simulink model "xEMU_SimulationModel3_rule1"  (R2017b)
settings: Solver=ode4  StartTime=0.0  StopTime=8192  FixedStep=0.01  RelTol=1e-3
undefined symbols (not defined in the file): a1, a2, a3, a4, ACO, BAT, Battery, DCT, DRT, EMS, ENV, Fahrzyklus_VS_modell, height_BAT, leistung, lib_bat, Maximum, Maximum_position, Num_cells, P_FC_max_long, P_FC_min_long, P_FC_step_max, Pbat_charge_max, Pbat_discharge_max, Pfc_max, Pfc_min, SOC_tar, time_peaks, TRM, velocity_peaks
libraries: simulink x5
(part 5 of 15)

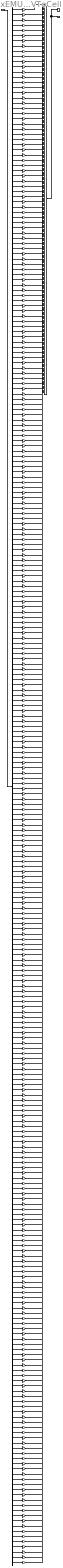
== system xEMU_SimulationModel3_rule1/Battery (BAT)_komplex/Subsystem/Thermal/FVToCell ==
  T_FV : Inport
  AddCell1 : Sum  Inputs=<binary blob, 300 chars, not shown>
  Demux : Demux  Outputs=300
  T_FV_{1..300} (300 alike) : Gain  Gain=0.0033333  SaturateOnIntegerOverflow=on  OutDataTypeStr=Inherit: Same as input  ParamDataTypeStr=Inherit: Same as input
  Out1 : Outport
  tag scope: T_CellElement1=global
  wires:
  T_FV/1 -> Demux/1
  Demux/1 -> T_FV_1/1
  Demux/2 -> T_FV_2/1
  Demux/3 -> T_FV_3/1
  Demux/4 -> T_FV_4/1
  Demux/5 -> T_FV_5/1
  Demux/6 -> T_FV_6/1
  Demux/7 -> T_FV_7/1
  Demux/8 -> T_FV_8/1
  Demux/9 -> T_FV_9/1
  Demux/10 -> T_FV_10/1
  Demux/11 -> T_FV_11/1
  Demux/12 -> T_FV_12/1
  Demux/13 -> T_FV_13/1
  Demux/14 -> T_FV_14/1
  Demux/15 -> T_FV_15/1
  Demux/16 -> T_FV_16/1
  Demux/17 -> T_FV_17/1
  Demux/18 -> T_FV_18/1
  Demux/19 -> T_FV_19/1
  Demux/20 -> T_FV_20/1
  Demux/21 -> T_FV_21/1
  Demux/22 -> T_FV_22/1
  Demux/23 -> T_FV_23/1
  Demux/24 -> T_FV_24/1
  Demux/25 -> T_FV_25/1
  Demux/26 -> T_FV_26/1
  Demux/27 -> T_FV_27/1
  Demux/28 -> T_FV_28/1
  Demux/29 -> T_FV_29/1
  Demux/30 -> T_FV_30/1
  Demux/31 -> T_FV_31/1
  Demux/32 -> T_FV_32/1
  Demux/33 -> T_FV_33/1
  Demux/34 -> T_FV_34/1
  Demux/35 -> T_FV_35/1
  Demux/36 -> T_FV_36/1
  Demux/37 -> T_FV_37/1
  Demux/38 -> T_FV_38/1
  Demux/39 -> T_FV_39/1
  Demux/40 -> T_FV_40/1
  Demux/41 -> T_FV_41/1
  Demux/42 -> T_FV_42/1
  Demux/43 -> T_FV_43/1
  Demux/44 -> T_FV_44/1
  Demux/45 -> T_FV_45/1
  Demux/46 -> T_FV_46/1
  Demux/47 -> T_FV_47/1
  Demux/48 -> T_FV_48/1
  Demux/49 -> T_FV_49/1
  Demux/50 -> T_FV_50/1
  Demux/51 -> T_FV_51/1
  Demux/52 -> T_FV_52/1
  Demux/53 -> T_FV_53/1
  Demux/54 -> T_FV_54/1
  Demux/55 -> T_FV_55/1
  Demux/56 -> T_FV_56/1
  Demux/57 -> T_FV_57/1
  Demux/58 -> T_FV_58/1
  Demux/59 -> T_FV_59/1
  Demux/60 -> T_FV_60/1
  Demux/61 -> T_FV_61/1
  Demux/62 -> T_FV_62/1
  Demux/63 -> T_FV_63/1
  Demux/64 -> T_FV_64/1
  Demux/65 -> T_FV_65/1
  Demux/66 -> T_FV_66/1
  Demux/67 -> T_FV_67/1
  Demux/68 -> T_FV_68/1
  Demux/69 -> T_FV_69/1
  Demux/70 -> T_FV_70/1
  Demux/71 -> T_FV_71/1
  Demux/72 -> T_FV_72/1
  Demux/73 -> T_FV_73/1
  Demux/74 -> T_FV_74/1
  Demux/75 -> T_FV_75/1
  Demux/76 -> T_FV_76/1
  Demux/77 -> T_FV_77/1
  Demux/78 -> T_FV_78/1
  Demux/79 -> T_FV_79/1
  Demux/80 -> T_FV_80/1
  Demux/81 -> T_FV_81/1
  Demux/82 -> T_FV_82/1
  Demux/83 -> T_FV_83/1
  Demux/84 -> T_FV_84/1
  Demux/85 -> T_FV_85/1
  Demux/86 -> T_FV_86/1
  Demux/87 -> T_FV_87/1
  Demux/88 -> T_FV_88/1
  Demux/89 -> T_FV_89/1
  Demux/90 -> T_FV_90/1
  Demux/91 -> T_FV_91/1
  Demux/92 -> T_FV_92/1
  Demux/93 -> T_FV_93/1
  Demux/94 -> T_FV_94/1
  Demux/95 -> T_FV_95/1
  Demux/96 -> T_FV_96/1
  Demux/97 -> T_FV_97/1
  Demux/98 -> T_FV_98/1
  Demux/99 -> T_FV_99/1
  Demux/100 -> T_FV_100/1
  Demux/101 -> T_FV_101/1
  Demux/102 -> T_FV_102/1
  Demux/103 -> T_FV_103/1
  Demux/104 -> T_FV_104/1
  Demux/105 -> T_FV_105/1
  Demux/106 -> T_FV_106/1
  Demux/107 -> T_FV_107/1
  Demux/108 -> T_FV_108/1
  Demux/109 -> T_FV_109/1
  Demux/110 -> T_FV_110/1
  Demux/111 -> T_FV_111/1
  Demux/112 -> T_FV_112/1
  Demux/113 -> T_FV_113/1
  Demux/114 -> T_FV_114/1
  Demux/115 -> T_FV_115/1
  Demux/116 -> T_FV_116/1
  Demux/117 -> T_FV_117/1
  Demux/118 -> T_FV_118/1
  Demux/119 -> T_FV_119/1
  Demux/120 -> T_FV_120/1
  Demux/121 -> T_FV_121/1
  Demux/122 -> T_FV_122/1
  Demux/123 -> T_FV_123/1
  Demux/124 -> T_FV_124/1
  Demux/125 -> T_FV_125/1
  Demux/126 -> T_FV_126/1
  Demux/127 -> T_FV_127/1
  Demux/128 -> T_FV_128/1
  Demux/129 -> T_FV_129/1
  Demux/130 -> T_FV_130/1
  Demux/131 -> T_FV_131/1
  Demux/132 -> T_FV_132/1
  Demux/133 -> T_FV_133/1
  Demux/134 -> T_FV_134/1
  Demux/135 -> T_FV_135/1
  Demux/136 -> T_FV_136/1
  Demux/137 -> T_FV_137/1
  Demux/138 -> T_FV_138/1
  Demux/139 -> T_FV_139/1
  Demux/140 -> T_FV_140/1
  Demux/141 -> T_FV_141/1
  Demux/142 -> T_FV_142/1
  Demux/143 -> T_FV_143/1
  Demux/144 -> T_FV_144/1
  Demux/145 -> T_FV_145/1
  Demux/146 -> T_FV_146/1
  Demux/147 -> T_FV_147/1
  Demux/148 -> T_FV_148/1
  Demux/149 -> T_FV_149/1
  Demux/150 -> T_FV_150/1
  Demux/151 -> T_FV_151/1
  Demux/152 -> T_FV_152/1
  Demux/153 -> T_FV_153/1
  Demux/154 -> T_FV_154/1
  Demux/155 -> T_FV_155/1
  Demux/156 -> T_FV_156/1
  Demux/157 -> T_FV_157/1
  Demux/158 -> T_FV_158/1
  Demux/159 -> T_FV_159/1
  Demux/160 -> T_FV_160/1
  Demux/161 -> T_FV_161/1
  Demux/162 -> T_FV_162/1
  Demux/163 -> T_FV_163/1
  Demux/164 -> T_FV_164/1
  Demux/165 -> T_FV_165/1
  Demux/166 -> T_FV_166/1
  Demux/167 -> T_FV_167/1
  Demux/168 -> T_FV_168/1
  Demux/169 -> T_FV_169/1
  Demux/170 -> T_FV_170/1
  Demux/171 -> T_FV_171/1
  Demux/172 -> T_FV_172/1
  Demux/173 -> T_FV_173/1
  Demux/174 -> T_FV_174/1
  Demux/175 -> T_FV_175/1
  Demux/176 -> T_FV_176/1
  Demux/177 -> T_FV_177/1
  Demux/178 -> T_FV_178/1
  Demux/179 -> T_FV_179/1
  Demux/180 -> T_FV_180/1
  Demux/181 -> T_FV_181/1
  Demux/182 -> T_FV_182/1
  Demux/183 -> T_FV_183/1
  Demux/184 -> T_FV_184/1
  Demux/185 -> T_FV_185/1
  Demux/186 -> T_FV_186/1
  Demux/187 -> T_FV_187/1
  Demux/188 -> T_FV_188/1
  Demux/189 -> T_FV_189/1
  Demux/190 -> T_FV_190/1
  Demux/191 -> T_FV_191/1
  Demux/192 -> T_FV_192/1
  Demux/193 -> T_FV_193/1
  Demux/194 -> T_FV_194/1
  Demux/195 -> T_FV_195/1
  Demux/196 -> T_FV_196/1
  Demux/197 -> T_FV_197/1
  Demux/198 -> T_FV_198/1
  Demux/199 -> T_FV_199/1
  Demux/200 -> T_FV_200/1
  Demux/201 -> T_FV_201/1
  Demux/202 -> T_FV_202/1
  Demux/203 -> T_FV_203/1
  Demux/204 -> T_FV_204/1
  Demux/205 -> T_FV_205/1
  Demux/206 -> T_FV_206/1
  Demux/207 -> T_FV_207/1
  Demux/208 -> T_FV_208/1
  Demux/209 -> T_FV_209/1
  Demux/210 -> T_FV_210/1
  Demux/211 -> T_FV_211/1
  Demux/212 -> T_FV_212/1
  Demux/213 -> T_FV_213/1
  Demux/214 -> T_FV_214/1
  Demux/215 -> T_FV_215/1
  Demux/216 -> T_FV_216/1
  Demux/217 -> T_FV_217/1
  Demux/218 -> T_FV_218/1
  Demux/219 -> T_FV_219/1
  Demux/220 -> T_FV_220/1
  Demux/221 -> T_FV_221/1
  Demux/222 -> T_FV_222/1
  Demux/223 -> T_FV_223/1
  Demux/224 -> T_FV_224/1
  Demux/225 -> T_FV_225/1
  Demux/226 -> T_FV_226/1
  Demux/227 -> T_FV_227/1
  Demux/228 -> T_FV_228/1
  Demux/229 -> T_FV_229/1
  Demux/230 -> T_FV_230/1
  Demux/231 -> T_FV_231/1
  Demux/232 -> T_FV_232/1
  Demux/233 -> T_FV_233/1
  Demux/234 -> T_FV_234/1
  Demux/235 -> T_FV_235/1
  Demux/236 -> T_FV_236/1
  Demux/237 -> T_FV_237/1
  Demux/238 -> T_FV_238/1
  Demux/239 -> T_FV_239/1
  Demux/240 -> T_FV_240/1
  Demux/241 -> T_FV_241/1
  Demux/242 -> T_FV_242/1
  Demux/243 -> T_FV_243/1
  Demux/244 -> T_FV_244/1
  Demux/245 -> T_FV_245/1
  Demux/246 -> T_FV_246/1
  Demux/247 -> T_FV_247/1
  Demux/248 -> T_FV_248/1
  Demux/249 -> T_FV_249/1
  Demux/250 -> T_FV_250/1
  Demux/251 -> T_FV_251/1
  Demux/252 -> T_FV_252/1
  Demux/253 -> T_FV_253/1
  Demux/254 -> T_FV_254/1
  Demux/255 -> T_FV_255/1
  Demux/256 -> T_FV_256/1
  Demux/257 -> T_FV_257/1
  Demux/258 -> T_FV_258/1
  Demux/259 -> T_FV_259/1
  Demux/260 -> T_FV_260/1
  Demux/261 -> T_FV_261/1
  Demux/262 -> T_FV_262/1
  Demux/263 -> T_FV_263/1
  Demux/264 -> T_FV_264/1
  Demux/265 -> T_FV_265/1
  Demux/266 -> T_FV_266/1
  Demux/267 -> T_FV_267/1
  Demux/268 -> T_FV_268/1
  Demux/269 -> T_FV_269/1
  Demux/270 -> T_FV_270/1
  Demux/271 -> T_FV_271/1
  Demux/272 -> T_FV_272/1
  Demux/273 -> T_FV_273/1
  Demux/274 -> T_FV_274/1
  Demux/275 -> T_FV_275/1
  Demux/276 -> T_FV_276/1
  Demux/277 -> T_FV_277/1
  Demux/278 -> T_FV_278/1
  Demux/279 -> T_FV_279/1
  Demux/280 -> T_FV_280/1
  Demux/281 -> T_FV_281/1
  Demux/282 -> T_FV_282/1
  Demux/283 -> T_FV_283/1
  Demux/284 -> T_FV_284/1
  Demux/285 -> T_FV_285/1
  Demux/286 -> T_FV_286/1
  Demux/287 -> T_FV_287/1
  Demux/288 -> T_FV_288/1
  Demux/289 -> T_FV_289/1
  Demux/290 -> T_FV_290/1
  Demux/291 -> T_FV_291/1
  Demux/292 -> T_FV_292/1
  Demux/293 -> T_FV_293/1
  Demux/294 -> T_FV_294/1
  Demux/295 -> T_FV_295/1
  Demux/296 -> T_FV_296/1
  Demux/297 -> T_FV_297/1
  Demux/298 -> T_FV_298/1
  Demux/299 -> T_FV_299/1
  Demux/300 -> T_FV_300/1
  AddCell1/1 -> Out1/1, [T_CellElement1]
  T_FV_1/1 -> AddCell1/1
  T_FV_2/1 -> AddCell1/2
  T_FV_3/1 -> AddCell1/3
  T_FV_4/1 -> AddCell1/4
  T_FV_5/1 -> AddCell1/5
  T_FV_6/1 -> AddCell1/6
  T_FV_7/1 -> AddCell1/7
  T_FV_8/1 -> AddCell1/8
  T_FV_9/1 -> AddCell1/9
  T_FV_10/1 -> AddCell1/10
  T_FV_11/1 -> AddCell1/11
  T_FV_12/1 -> AddCell1/12
  T_FV_13/1 -> AddCell1/13
  T_FV_14/1 -> AddCell1/14
  T_FV_15/1 -> AddCell1/15
  T_FV_16/1 -> AddCell1/16
  T_FV_17/1 -> AddCell1/17
  T_FV_18/1 -> AddCell1/18
  T_FV_19/1 -> AddCell1/19
  T_FV_20/1 -> AddCell1/20
  T_FV_21/1 -> AddCell1/21
  T_FV_22/1 -> AddCell1/22
  T_FV_23/1 -> AddCell1/23
  T_FV_24/1 -> AddCell1/24
  T_FV_25/1 -> AddCell1/25
  T_FV_26/1 -> AddCell1/26
  T_FV_27/1 -> AddCell1/27
  T_FV_28/1 -> AddCell1/28
  T_FV_29/1 -> AddCell1/29
  T_FV_30/1 -> AddCell1/30
  T_FV_31/1 -> AddCell1/31
  T_FV_32/1 -> AddCell1/32
  T_FV_33/1 -> AddCell1/33
  T_FV_34/1 -> AddCell1/34
  T_FV_35/1 -> AddCell1/35
  T_FV_36/1 -> AddCell1/36
  T_FV_37/1 -> AddCell1/37
  T_FV_38/1 -> AddCell1/38
  T_FV_39/1 -> AddCell1/39
  T_FV_40/1 -> AddCell1/40
  T_FV_41/1 -> AddCell1/41
  T_FV_42/1 -> AddCell1/42
  T_FV_43/1 -> AddCell1/43
  T_FV_44/1 -> AddCell1/44
  T_FV_45/1 -> AddCell1/45
  T_FV_46/1 -> AddCell1/46
  T_FV_47/1 -> AddCell1/47
  T_FV_48/1 -> AddCell1/48
  T_FV_49/1 -> AddCell1/49
  T_FV_50/1 -> AddCell1/50
  T_FV_51/1 -> AddCell1/51
  T_FV_52/1 -> AddCell1/52
  T_FV_53/1 -> AddCell1/53
  T_FV_54/1 -> AddCell1/54
  T_FV_55/1 -> AddCell1/55
  T_FV_56/1 -> AddCell1/56
  T_FV_57/1 -> AddCell1/57
  T_FV_58/1 -> AddCell1/58
  T_FV_59/1 -> AddCell1/59
  T_FV_60/1 -> AddCell1/60
  T_FV_61/1 -> AddCell1/61
  T_FV_62/1 -> AddCell1/62
  T_FV_63/1 -> AddCell1/63
  T_FV_64/1 -> AddCell1/64
  T_FV_65/1 -> AddCell1/65
  T_FV_66/1 -> AddCell1/66
  T_FV_67/1 -> AddCell1/67
  T_FV_68/1 -> AddCell1/68
  T_FV_69/1 -> AddCell1/69
  T_FV_70/1 -> AddCell1/70
  T_FV_71/1 -> AddCell1/71
  T_FV_72/1 -> AddCell1/72
  T_FV_73/1 -> AddCell1/73
  T_FV_74/1 -> AddCell1/74
  T_FV_75/1 -> AddCell1/75
  T_FV_76/1 -> AddCell1/76
  T_FV_77/1 -> AddCell1/77
  T_FV_78/1 -> AddCell1/78
  T_FV_79/1 -> AddCell1/79
  T_FV_80/1 -> AddCell1/80
  T_FV_81/1 -> AddCell1/81
  T_FV_82/1 -> AddCell1/82
  T_FV_83/1 -> AddCell1/83
  T_FV_84/1 -> AddCell1/84
  T_FV_85/1 -> AddCell1/85
  T_FV_86/1 -> AddCell1/86
  T_FV_87/1 -> AddCell1/87
  T_FV_88/1 -> AddCell1/88
  T_FV_89/1 -> AddCell1/89
  T_FV_90/1 -> AddCell1/90
  T_FV_91/1 -> AddCell1/91
  T_FV_92/1 -> AddCell1/92
  T_FV_93/1 -> AddCell1/93
  T_FV_94/1 -> AddCell1/94
  T_FV_95/1 -> AddCell1/95
  T_FV_96/1 -> AddCell1/96
  T_FV_97/1 -> AddCell1/97
  T_FV_98/1 -> AddCell1/98
  T_FV_99/1 -> AddCell1/99
  T_FV_100/1 -> AddCell1/100
  T_FV_101/1 -> AddCell1/101
  T_FV_102/1 -> AddCell1/102
  T_FV_103/1 -> AddCell1/103
  T_FV_104/1 -> AddCell1/104
  T_FV_105/1 -> AddCell1/105
  T_FV_106/1 -> AddCell1/106
  T_FV_107/1 -> AddCell1/107
  T_FV_108/1 -> AddCell1/108
  T_FV_109/1 -> AddCell1/109
  T_FV_110/1 -> AddCell1/110
  T_FV_111/1 -> AddCell1/111
  T_FV_112/1 -> AddCell1/112
  T_FV_113/1 -> AddCell1/113
  T_FV_114/1 -> AddCell1/114
  T_FV_115/1 -> AddCell1/115
  T_FV_116/1 -> AddCell1/116
  T_FV_117/1 -> AddCell1/117
  T_FV_118/1 -> AddCell1/118
  T_FV_119/1 -> AddCell1/119
  T_FV_120/1 -> AddCell1/120
  T_FV_121/1 -> AddCell1/121
  T_FV_122/1 -> AddCell1/122
  T_FV_123/1 -> AddCell1/123
  T_FV_124/1 -> AddCell1/124
  T_FV_125/1 -> AddCell1/125
  T_FV_126/1 -> AddCell1/126
  T_FV_127/1 -> AddCell1/127
  T_FV_128/1 -> AddCell1/128
  T_FV_129/1 -> AddCell1/129
  T_FV_130/1 -> AddCell1/130
  T_FV_131/1 -> AddCell1/131
  T_FV_132/1 -> AddCell1/132
  T_FV_133/1 -> AddCell1/133
  T_FV_134/1 -> AddCell1/134
  T_FV_135/1 -> AddCell1/135
  T_FV_136/1 -> AddCell1/136
  T_FV_137/1 -> AddCell1/137
  T_FV_138/1 -> AddCell1/138
  T_FV_139/1 -> AddCell1/139
  T_FV_140/1 -> AddCell1/140
  T_FV_141/1 -> AddCell1/141
  T_FV_142/1 -> AddCell1/142
  T_FV_143/1 -> AddCell1/143
  T_FV_144/1 -> AddCell1/144
  T_FV_145/1 -> AddCell1/145
  T_FV_146/1 -> AddCell1/146
  T_FV_147/1 -> AddCell1/147
  T_FV_148/1 -> AddCell1/148
  T_FV_149/1 -> AddCell1/149
  T_FV_150/1 -> AddCell1/150
  T_FV_151/1 -> AddCell1/151
  T_FV_152/1 -> AddCell1/152
  T_FV_153/1 -> AddCell1/153
  T_FV_154/1 -> AddCell1/154
  T_FV_155/1 -> AddCell1/155
  T_FV_156/1 -> AddCell1/156
  T_FV_157/1 -> AddCell1/157
  T_FV_158/1 -> AddCell1/158
  T_FV_159/1 -> AddCell1/159
  T_FV_160/1 -> AddCell1/160
  T_FV_161/1 -> AddCell1/161
  T_FV_162/1 -> AddCell1/162
  T_FV_163/1 -> AddCell1/163
  T_FV_164/1 -> AddCell1/164
  T_FV_165/1 -> AddCell1/165
  T_FV_166/1 -> AddCell1/166
  T_FV_167/1 -> AddCell1/167
  T_FV_168/1 -> AddCell1/168
  T_FV_169/1 -> AddCell1/169
  T_FV_170/1 -> AddCell1/170
  T_FV_171/1 -> AddCell1/171
  T_FV_172/1 -> AddCell1/172
  T_FV_173/1 -> AddCell1/173
  T_FV_174/1 -> AddCell1/174
  T_FV_175/1 -> AddCell1/175
  T_FV_176/1 -> AddCell1/176
  T_FV_177/1 -> AddCell1/177
  T_FV_178/1 -> AddCell1/178
  T_FV_179/1 -> AddCell1/179
  T_FV_180/1 -> AddCell1/180
  T_FV_181/1 -> AddCell1/181
  T_FV_182/1 -> AddCell1/182
  T_FV_183/1 -> AddCell1/183
  T_FV_184/1 -> AddCell1/184
  T_FV_185/1 -> AddCell1/185
  T_FV_186/1 -> AddCell1/186
  T_FV_187/1 -> AddCell1/187
  T_FV_188/1 -> AddCell1/188
  T_FV_189/1 -> AddCell1/189
  T_FV_190/1 -> AddCell1/190
  T_FV_191/1 -> AddCell1/191
  T_FV_192/1 -> AddCell1/192
  T_FV_193/1 -> AddCell1/193
  T_FV_194/1 -> AddCell1/194
  T_FV_195/1 -> AddCell1/195
  T_FV_196/1 -> AddCell1/196
  T_FV_197/1 -> AddCell1/197
  T_FV_198/1 -> AddCell1/198
  T_FV_199/1 -> AddCell1/199
  T_FV_200/1 -> AddCell1/200
  T_FV_201/1 -> AddCell1/201
  T_FV_202/1 -> AddCell1/202
  T_FV_203/1 -> AddCell1/203
  T_FV_204/1 -> AddCell1/204
  T_FV_205/1 -> AddCell1/205
  T_FV_206/1 -> AddCell1/206
  T_FV_207/1 -> AddCell1/207
  T_FV_208/1 -> AddCell1/208
  T_FV_209/1 -> AddCell1/209
  T_FV_210/1 -> AddCell1/210
  T_FV_211/1 -> AddCell1/211
  T_FV_212/1 -> AddCell1/212
  T_FV_213/1 -> AddCell1/213
  T_FV_214/1 -> AddCell1/214
  T_FV_215/1 -> AddCell1/215
  T_FV_216/1 -> AddCell1/216
  T_FV_217/1 -> AddCell1/217
  T_FV_218/1 -> AddCell1/218
  T_FV_219/1 -> AddCell1/219
  T_FV_220/1 -> AddCell1/220
  T_FV_221/1 -> AddCell1/221
  T_FV_222/1 -> AddCell1/222
  T_FV_223/1 -> AddCell1/223
  T_FV_224/1 -> AddCell1/224
  T_FV_225/1 -> AddCell1/225
  T_FV_226/1 -> AddCell1/226
  T_FV_227/1 -> AddCell1/227
  T_FV_228/1 -> AddCell1/228
  T_FV_229/1 -> AddCell1/229
  T_FV_230/1 -> AddCell1/230
  T_FV_231/1 -> AddCell1/231
  T_FV_232/1 -> AddCell1/232
  T_FV_233/1 -> AddCell1/233
  T_FV_234/1 -> AddCell1/234
  T_FV_235/1 -> AddCell1/235
  T_FV_236/1 -> AddCell1/236
  T_FV_237/1 -> AddCell1/237
  T_FV_238/1 -> AddCell1/238
  T_FV_239/1 -> AddCell1/239
  T_FV_240/1 -> AddCell1/240
  T_FV_241/1 -> AddCell1/241
  T_FV_242/1 -> AddCell1/242
  T_FV_243/1 -> AddCell1/243
  T_FV_244/1 -> AddCell1/244
  T_FV_245/1 -> AddCell1/245
  T_FV_246/1 -> AddCell1/246
  T_FV_247/1 -> AddCell1/247
  T_FV_248/1 -> AddCell1/248
  T_FV_249/1 -> AddCell1/249
  T_FV_250/1 -> AddCell1/250
  T_FV_251/1 -> AddCell1/251
  T_FV_252/1 -> AddCell1/252
  T_FV_253/1 -> AddCell1/253
  T_FV_254/1 -> AddCell1/254
  T_FV_255/1 -> AddCell1/255
  T_FV_256/1 -> AddCell1/256
  T_FV_257/1 -> AddCell1/257
  T_FV_258/1 -> AddCell1/258
  T_FV_259/1 -> AddCell1/259
  T_FV_260/1 -> AddCell1/260
  T_FV_261/1 -> AddCell1/261
  T_FV_262/1 -> AddCell1/262
  T_FV_263/1 -> AddCell1/263
  T_FV_264/1 -> AddCell1/264
  T_FV_265/1 -> AddCell1/265
  T_FV_266/1 -> AddCell1/266
  T_FV_267/1 -> AddCell1/267
  T_FV_268/1 -> AddCell1/268
  T_FV_269/1 -> AddCell1/269
  T_FV_270/1 -> AddCell1/270
  T_FV_271/1 -> AddCell1/271
  T_FV_272/1 -> AddCell1/272
  T_FV_273/1 -> AddCell1/273
  T_FV_274/1 -> AddCell1/274
  T_FV_275/1 -> AddCell1/275
  T_FV_276/1 -> AddCell1/276
  T_FV_277/1 -> AddCell1/277
  T_FV_278/1 -> AddCell1/278
  T_FV_279/1 -> AddCell1/279
  T_FV_280/1 -> AddCell1/280
  T_FV_281/1 -> AddCell1/281
  T_FV_282/1 -> AddCell1/282
  T_FV_283/1 -> AddCell1/283
  T_FV_284/1 -> AddCell1/284
  T_FV_285/1 -> AddCell1/285
  T_FV_286/1 -> AddCell1/286
  T_FV_287/1 -> AddCell1/287
  T_FV_288/1 -> AddCell1/288
  T_FV_289/1 -> AddCell1/289
  T_FV_290/1 -> AddCell1/290
  T_FV_291/1 -> AddCell1/291
  T_FV_292/1 -> AddCell1/292
  T_FV_293/1 -> AddCell1/293
  T_FV_294/1 -> AddCell1/294
  T_FV_295/1 -> AddCell1/295
  T_FV_296/1 -> AddCell1/296
  T_FV_297/1 -> AddCell1/297
  T_FV_298/1 -> AddCell1/298
  T_FV_299/1 -> AddCell1/299
  T_FV_300/1 -> AddCell1/300

== system xEMU_SimulationModel3_rule1/Battery (BAT)_mittel/Battery/CellCurrentMatrices/Component0 ==
  ColConst : Constant  Value=0
  RowConst : Constant  Value=0
  Row : Outport
  Col : Outport  Port=2
  Value : Outport  Port=3
  wires:
  ColConst/1 -> Col/1
  RowConst/1 -> Row/1
  [InputCurrent] -> Value/1

== system xEMU_SimulationModel3_rule1/Battery (BAT)_mittel/Battery/CellCurrentMatrices/Component1 ==
  ColConst : Constant  Value=0
  RowConst : Constant  Value=0
  Row : Outport
  Col : Outport  Port=2
  Value : Outport  Port=3
  wires:
  ColConst/1 -> Col/1
  RowConst/1 -> Row/1
  [InputCurrent] -> Value/1

== system xEMU_SimulationModel3_rule1/Battery (BAT)_mittel/Battery/CellVoltageMatrices/Component0 ==
  Add2_1 : Sum
  Add3_1 : Sum
  Add3_2 : Sum
  Add4_1 : Sum
  ColConst : Constant  Value=0
  Mul2_3 : Product
  RowConst : Constant  Value=0
  Row : Outport
  Col : Outport  Port=2
  Value : Outport  Port=3
  wires:
  ColConst/1 -> Col/1
  RowConst/1 -> Row/1
  Add4_1/1 -> Value/1
  Add3_1/1 -> Add4_1/1
  Add2_1/1 -> Add3_1/1
  [State1] -> Add2_1/1
  [State2] -> Add2_1/2
  [State3] -> Add3_1/2
  Add3_2/1 -> Add4_1/2
  Mul2_3/1 -> Add3_2/1
  [InputCurrent] -> Mul2_3/1
  [ID2_ObjR] -> Mul2_3/2
  [ID6_ObjV] -> Add3_2/2

== system xEMU_SimulationModel3_rule1/Battery (BAT)_mittel/Battery/CellVoltageMatrices/Component1 ==
  Add2_1 : Sum
  Add3_1 : Sum
  Add3_2 : Sum
  Add4_1 : Sum
  ColConst : Constant  Value=0
  Mul2_3 : Product
  RowConst : Constant  Value=0
  Row : Outport
  Col : Outport  Port=2
  Value : Outport  Port=3
  wires:
  ColConst/1 -> Col/1
  RowConst/1 -> Row/1
  Add4_1/1 -> Value/1
  Add3_1/1 -> Add4_1/1
  Add2_1/1 -> Add3_1/1
  [State1] -> Add2_1/1
  [State2] -> Add2_1/2
  [State3] -> Add3_1/2
  Add3_2/1 -> Add4_1/2
  Mul2_3/1 -> Add3_2/1
  [InputCurrent] -> Mul2_3/1
  [ID2_ObjR] -> Mul2_3/2
  [ID6_ObjV] -> Add3_2/2

== system xEMU_SimulationModel3_rule1/Battery (BAT)_mittel/Battery/ElectricalCircuit/SerialTwoPort_Elem1 ==
  Cellelement_Elem1 : Subsystem

== system xEMU_SimulationModel3_rule1/Battery (BAT)_mittel/Battery/MatrixAxC/StateComponent0 ==
  Add5_1 : Sum
  ColConst : Constant  Value=0
  Const1_1 : Constant  Value=1.000000
  Div2_1 : Product  Inputs=*/
  Div4_2 : Product  Inputs=*/
  Integrator : Integrator
  Mul3_3 : Product
  Mul4_1 : Product
  Neg3_2 : Gain  Gain=-1
  RowConst : Constant  Value=0
  Row : Outport
  Col : Outport  Port=2
  tag scope: State1=scoped
  wires:
  Integrator/1 -> [State1]
  ColConst/1 -> Col/1
  RowConst/1 -> Row/1
  Add5_1/1 -> Integrator/1
  Mul4_1/1 -> Add5_1/1
  [State1] -> Mul4_1/1
  Neg3_2/1 -> Mul4_1/2
  Div2_1/1 -> Neg3_2/1
  Const1_1/1 -> Div2_1/1
  [ID3_ObjTau] -> Div2_1/2
  Div4_2/1 -> Add5_1/2
  Mul3_3/1 -> Div4_2/1
  [InputCurrent] -> Mul3_3/1
  [ID3_ObjR] -> Mul3_3/2
  [ID3_ObjTau] -> Div4_2/2

== system xEMU_SimulationModel3_rule1/Battery (BAT)_mittel/Battery/MatrixAxC/StateComponent1 ==
  Add5_1 : Sum
  ColConst : Constant  Value=0
  Const1_1 : Constant  Value=1.000000
  Div2_1 : Product  Inputs=*/
  Div4_2 : Product  Inputs=*/
  Integrator : Integrator
  Mul3_3 : Product
  Mul4_1 : Product
  Neg3_2 : Gain  Gain=-1
  RowConst : Constant
  Row : Outport
  Col : Outport  Port=2
  tag scope: State2=scoped
  wires:
  Integrator/1 -> [State2]
  ColConst/1 -> Col/1
  RowConst/1 -> Row/1
  Add5_1/1 -> Integrator/1
  Mul4_1/1 -> Add5_1/1
  [State2] -> Mul4_1/1
  Neg3_2/1 -> Mul4_1/2
  Div2_1/1 -> Neg3_2/1
  Const1_1/1 -> Div2_1/1
  [ID4_ObjTau] -> Div2_1/2
  Div4_2/1 -> Add5_1/2
  Mul3_3/1 -> Div4_2/1
  [InputCurrent] -> Mul3_3/1
  [ID4_ObjR] -> Mul3_3/2
  [ID4_ObjTau] -> Div4_2/2

== system xEMU_SimulationModel3_rule1/Battery (BAT)_mittel/Battery/MatrixAxC/StateComponent2 ==
  Add5_1 : Sum
  ColConst : Constant  Value=0
  Const1_1 : Constant  Value=1.000000
  Div2_1 : Product  Inputs=*/
  Div4_2 : Product  Inputs=*/
  Integrator : Integrator
  Mul3_3 : Product
  Mul4_1 : Product
  Neg3_2 : Gain  Gain=-1
  RowConst : Constant  Value=2
  Row : Outport
  Col : Outport  Port=2
  tag scope: State3=scoped
  wires:
  Integrator/1 -> [State3]
  ColConst/1 -> Col/1
  RowConst/1 -> Row/1
  Add5_1/1 -> Integrator/1
  Mul4_1/1 -> Add5_1/1
  [State3] -> Mul4_1/1
  Neg3_2/1 -> Mul4_1/2
  Div2_1/1 -> Neg3_2/1
  Const1_1/1 -> Div2_1/1
  [ID5_ObjTau] -> Div2_1/2
  Div4_2/1 -> Add5_1/2
  Mul3_3/1 -> Div4_2/1
  [InputCurrent] -> Mul3_3/1
  [ID5_ObjR] -> Mul3_3/2
  [ID5_ObjTau] -> Div4_2/2

== system xEMU_SimulationModel3_rule1/Battery (BAT)_mittel/Battery/PowerMatrix/Component0 ==
  Add4_1 : Sum
  Add5_1 : Sum
  Add6_1 : Sum
  ColConst : Constant  Value=0
  Div3_1 : Product  Inputs=*/
  Div3_2 : Product  Inputs=*/
  Div4_2 : Product  Inputs=*/
  Mul5_2 : Product
  RowConst : Constant  Value=0
  Squ2_1 : Math  Operator=square  SaturateOnIntegerOverflow=on
  Squ2_3 : Math  Operator=square  SaturateOnIntegerOverflow=on
  Squ3_3 : Math  Operator=square  SaturateOnIntegerOverflow=on
  Squ4_3 : Math  Operator=square  SaturateOnIntegerOverflow=on
  Row : Outport
  Col : Outport  Port=2
  Value : Outport  Port=3
  wires:
  ColConst/1 -> Col/1
  RowConst/1 -> Row/1
  Add6_1/1 -> Value/1
  Add5_1/1 -> Add6_1/1
  Add4_1/1 -> Add5_1/1
  Div3_1/1 -> Add4_1/1
  Squ2_1/1 -> Div3_1/1
  [State1] -> Squ2_1/1
  [ID3_ObjR] -> Div3_1/2
  Div3_2/1 -> Add4_1/2
  Squ2_3/1 -> Div3_2/1
  [State2] -> Squ2_3/1
  [ID4_ObjR] -> Div3_2/2
  Div4_2/1 -> Add5_1/2
  Squ3_3/1 -> Div4_2/1
  [State3] -> Squ3_3/1
  [ID5_ObjR] -> Div4_2/2
  Mul5_2/1 -> Add6_1/2
  Squ4_3/1 -> Mul5_2/1
  [InputCurrent] -> Squ4_3/1
  [ID2_ObjR] -> Mul5_2/2

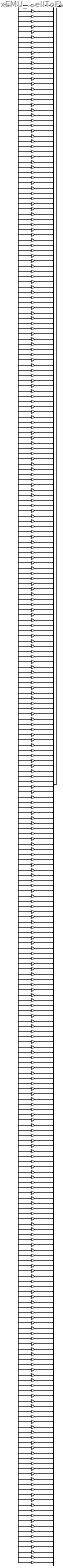
== system xEMU_SimulationModel3_rule1/Battery (BAT)_mittel/Battery/Thermal/CellToFV ==
  Mux : Mux  Inputs=300
  P_FV_{1..300} (300 alike) : Gain  Gain=0.0033333  SaturateOnIntegerOverflow=on  OutDataTypeStr=Inherit: Same as input  ParamDataTypeStr=Inherit: Same as input
  P_FV : Outport
  wires:
  Mux/1 -> P_FV/1
  [P_CellElement1] -> P_FV_1/1, P_FV_2/1, P_FV_3/1, P_FV_4/1, P_FV_5/1, P_FV_6/1, P_FV_7/1, P_FV_8/1, P_FV_9/1, P_FV_10/1, P_FV_11/1, P_FV_12/1, P_FV_13/1, P_FV_14/1, P_FV_15/1, P_FV_16/1, P_FV_17/1, P_FV_18/1, P_FV_19/1, P_FV_20/1, P_FV_21/1, P_FV_22/1, P_FV_23/1, P_FV_24/1, P_FV_25/1, P_FV_26/1, P_FV_27/1, P_FV_28/1, P_FV_29/1, P_FV_30/1, P_FV_31/1, P_FV_32/1, P_FV_33/1, P_FV_34/1, P_FV_35/1, P_FV_36/1, P_FV_37/1, P_FV_38/1, P_FV_39/1, P_FV_40/1, P_FV_41/1, P_FV_42/1, P_FV_43/1, P_FV_44/1, P_FV_45/1, P_FV_46/1, P_FV_47/1, P_FV_48/1, P_FV_49/1, P_FV_50/1, P_FV_51/1, P_FV_52/1, P_FV_53/1, P_FV_54/1, P_FV_55/1, P_FV_56/1, P_FV_57/1, P_FV_58/1, P_FV_59/1, P_FV_60/1, P_FV_61/1, P_FV_62/1, P_FV_63/1, P_FV_64/1, P_FV_65/1, P_FV_66/1, P_FV_67/1, P_FV_68/1, P_FV_69/1, P_FV_70/1, P_FV_71/1, P_FV_72/1, P_FV_73/1, P_FV_74/1, P_FV_75/1, P_FV_76/1, P_FV_77/1, P_FV_78/1, P_FV_79/1, P_FV_80/1, P_FV_81/1, P_FV_82/1, P_FV_83/1, P_FV_84/1, P_FV_85/1, P_FV_86/1, P_FV_87/1, P_FV_88/1, P_FV_89/1, P_FV_90/1, P_FV_91/1, P_FV_92/1, P_FV_93/1, P_FV_94/1, P_FV_95/1, P_FV_96/1, P_FV_97/1, P_FV_98/1, P_FV_99/1, P_FV_100/1, P_FV_101/1, P_FV_102/1, P_FV_103/1, P_FV_104/1, P_FV_105/1, P_FV_106/1, P_FV_107/1, P_FV_108/1, P_FV_109/1, P_FV_110/1, P_FV_111/1, P_FV_112/1, P_FV_113/1, P_FV_114/1, P_FV_115/1, P_FV_116/1, P_FV_117/1, P_FV_118/1, P_FV_119/1, P_FV_120/1, P_FV_121/1, P_FV_122/1, P_FV_123/1, P_FV_124/1, P_FV_125/1, P_FV_126/1, P_FV_127/1, P_FV_128/1, P_FV_129/1, P_FV_130/1, P_FV_131/1, P_FV_132/1, P_FV_133/1, P_FV_134/1, P_FV_135/1, P_FV_136/1, P_FV_137/1, P_FV_138/1, P_FV_139/1, P_FV_140/1, P_FV_141/1, P_FV_142/1, P_FV_143/1, P_FV_144/1, P_FV_145/1, P_FV_146/1, P_FV_147/1, P_FV_148/1, P_FV_149/1, P_FV_150/1, P_FV_151/1, P_FV_152/1, P_FV_153/1, P_FV_154/1, P_FV_155/1, P_FV_156/1, P_FV_157/1, P_FV_158/1, P_FV_159/1, P_FV_160/1, P_FV_161/1, P_FV_162/1, P_FV_163/1, P_FV_164/1, P_FV_165/1, P_FV_166/1, P_FV_167/1, P_FV_168/1, P_FV_169/1, P_FV_170/1, P_FV_171/1, P_FV_172/1, P_FV_173/1, P_FV_174/1, P_FV_175/1, P_FV_176/1, P_FV_177/1, P_FV_178/1, P_FV_179/1, P_FV_180/1, P_FV_181/1, P_FV_182/1, P_FV_183/1, P_FV_184/1, P_FV_185/1, P_FV_186/1, P_FV_187/1, P_FV_188/1, P_FV_189/1, P_FV_190/1, P_FV_191/1, P_FV_192/1, P_FV_193/1, P_FV_194/1, P_FV_195/1, P_FV_196/1, P_FV_197/1, P_FV_198/1, P_FV_199/1, P_FV_200/1, P_FV_201/1, P_FV_202/1, P_FV_203/1, P_FV_204/1, P_FV_205/1, P_FV_206/1, P_FV_207/1, P_FV_208/1, P_FV_209/1, P_FV_210/1, P_FV_211/1, P_FV_212/1, P_FV_213/1, P_FV_214/1, P_FV_215/1, P_FV_216/1, P_FV_217/1, P_FV_218/1, P_FV_219/1, P_FV_220/1, P_FV_221/1, P_FV_222/1, P_FV_223/1, P_FV_224/1, P_FV_225/1, P_FV_226/1, P_FV_227/1, P_FV_228/1, P_FV_229/1, P_FV_230/1, P_FV_231/1, P_FV_232/1, P_FV_233/1, P_FV_234/1, P_FV_235/1, P_FV_236/1, P_FV_237/1, P_FV_238/1, P_FV_239/1, P_FV_240/1, P_FV_241/1, P_FV_242/1, P_FV_243/1, P_FV_244/1, P_FV_245/1, P_FV_246/1, P_FV_247/1, P_FV_248/1, P_FV_249/1, P_FV_250/1, P_FV_251/1, P_FV_252/1, P_FV_253/1, P_FV_254/1, P_FV_255/1, P_FV_256/1, P_FV_257/1, P_FV_258/1, P_FV_259/1, P_FV_260/1, P_FV_261/1, P_FV_262/1, P_FV_263/1, P_FV_264/1, P_FV_265/1, P_FV_266/1, P_FV_267/1, P_FV_268/1, P_FV_269/1, P_FV_270/1, P_FV_271/1, P_FV_272/1, P_FV_273/1, P_FV_274/1, P_FV_275/1, P_FV_276/1, P_FV_277/1, P_FV_278/1, P_FV_279/1, P_FV_280/1, P_FV_281/1, P_FV_282/1, P_FV_283/1, P_FV_284/1, P_FV_285/1, P_FV_286/1, P_FV_287/1, P_FV_288/1, P_FV_289/1, P_FV_290/1, P_FV_291/1, P_FV_292/1, P_FV_293/1, P_FV_294/1, P_FV_295/1, P_FV_296/1, P_FV_297/1, P_FV_298/1, P_FV_299/1, P_FV_300/1
  P_FV_1/1 -> Mux/1
  P_FV_2/1 -> Mux/2
  P_FV_3/1 -> Mux/3
  P_FV_4/1 -> Mux/4
  P_FV_5/1 -> Mux/5
  P_FV_6/1 -> Mux/6
  P_FV_7/1 -> Mux/7
  P_FV_8/1 -> Mux/8
  P_FV_9/1 -> Mux/9
  P_FV_10/1 -> Mux/10
  P_FV_11/1 -> Mux/11
  P_FV_12/1 -> Mux/12
  P_FV_13/1 -> Mux/13
  P_FV_14/1 -> Mux/14
  P_FV_15/1 -> Mux/15
  P_FV_16/1 -> Mux/16
  P_FV_17/1 -> Mux/17
  P_FV_18/1 -> Mux/18
  P_FV_19/1 -> Mux/19
  P_FV_20/1 -> Mux/20
  P_FV_21/1 -> Mux/21
  P_FV_22/1 -> Mux/22
  P_FV_23/1 -> Mux/23
  P_FV_24/1 -> Mux/24
  P_FV_25/1 -> Mux/25
  P_FV_26/1 -> Mux/26
  P_FV_27/1 -> Mux/27
  P_FV_28/1 -> Mux/28
  P_FV_29/1 -> Mux/29
  P_FV_30/1 -> Mux/30
  P_FV_31/1 -> Mux/31
  P_FV_32/1 -> Mux/32
  P_FV_33/1 -> Mux/33
  P_FV_34/1 -> Mux/34
  P_FV_35/1 -> Mux/35
  P_FV_36/1 -> Mux/36
  P_FV_37/1 -> Mux/37
  P_FV_38/1 -> Mux/38
  P_FV_39/1 -> Mux/39
  P_FV_40/1 -> Mux/40
  P_FV_41/1 -> Mux/41
  P_FV_42/1 -> Mux/42
  P_FV_43/1 -> Mux/43
  P_FV_44/1 -> Mux/44
  P_FV_45/1 -> Mux/45
  P_FV_46/1 -> Mux/46
  P_FV_47/1 -> Mux/47
  P_FV_48/1 -> Mux/48
  P_FV_49/1 -> Mux/49
  P_FV_50/1 -> Mux/50
  P_FV_51/1 -> Mux/51
  P_FV_52/1 -> Mux/52
  P_FV_53/1 -> Mux/53
  P_FV_54/1 -> Mux/54
  P_FV_55/1 -> Mux/55
  P_FV_56/1 -> Mux/56
  P_FV_57/1 -> Mux/57
  P_FV_58/1 -> Mux/58
  P_FV_59/1 -> Mux/59
  P_FV_60/1 -> Mux/60
  P_FV_61/1 -> Mux/61
  P_FV_62/1 -> Mux/62
  P_FV_63/1 -> Mux/63
  P_FV_64/1 -> Mux/64
  P_FV_65/1 -> Mux/65
  P_FV_66/1 -> Mux/66
  P_FV_67/1 -> Mux/67
  P_FV_68/1 -> Mux/68
  P_FV_69/1 -> Mux/69
  P_FV_70/1 -> Mux/70
  P_FV_71/1 -> Mux/71
  P_FV_72/1 -> Mux/72
  P_FV_73/1 -> Mux/73
  P_FV_74/1 -> Mux/74
  P_FV_75/1 -> Mux/75
  P_FV_76/1 -> Mux/76
  P_FV_77/1 -> Mux/77
  P_FV_78/1 -> Mux/78
  P_FV_79/1 -> Mux/79
  P_FV_80/1 -> Mux/80
  P_FV_81/1 -> Mux/81
  P_FV_82/1 -> Mux/82
  P_FV_83/1 -> Mux/83
  P_FV_84/1 -> Mux/84
  P_FV_85/1 -> Mux/85
  P_FV_86/1 -> Mux/86
  P_FV_87/1 -> Mux/87
  P_FV_88/1 -> Mux/88
  P_FV_89/1 -> Mux/89
  P_FV_90/1 -> Mux/90
  P_FV_91/1 -> Mux/91
  P_FV_92/1 -> Mux/92
  P_FV_93/1 -> Mux/93
  P_FV_94/1 -> Mux/94
  P_FV_95/1 -> Mux/95
  P_FV_96/1 -> Mux/96
  P_FV_97/1 -> Mux/97
  P_FV_98/1 -> Mux/98
  P_FV_99/1 -> Mux/99
  P_FV_100/1 -> Mux/100
  P_FV_101/1 -> Mux/101
  P_FV_102/1 -> Mux/102
  P_FV_103/1 -> Mux/103
  P_FV_104/1 -> Mux/104
  P_FV_105/1 -> Mux/105
  P_FV_106/1 -> Mux/106
  P_FV_107/1 -> Mux/107
  P_FV_108/1 -> Mux/108
  P_FV_109/1 -> Mux/109
  P_FV_110/1 -> Mux/110
  P_FV_111/1 -> Mux/111
  P_FV_112/1 -> Mux/112
  P_FV_113/1 -> Mux/113
  P_FV_114/1 -> Mux/114
  P_FV_115/1 -> Mux/115
  P_FV_116/1 -> Mux/116
  P_FV_117/1 -> Mux/117
  P_FV_118/1 -> Mux/118
  P_FV_119/1 -> Mux/119
  P_FV_120/1 -> Mux/120
  P_FV_121/1 -> Mux/121
  P_FV_122/1 -> Mux/122
  P_FV_123/1 -> Mux/123
  P_FV_124/1 -> Mux/124
  P_FV_125/1 -> Mux/125
  P_FV_126/1 -> Mux/126
  P_FV_127/1 -> Mux/127
  P_FV_128/1 -> Mux/128
  P_FV_129/1 -> Mux/129
  P_FV_130/1 -> Mux/130
  P_FV_131/1 -> Mux/131
  P_FV_132/1 -> Mux/132
  P_FV_133/1 -> Mux/133
  P_FV_134/1 -> Mux/134
  P_FV_135/1 -> Mux/135
  P_FV_136/1 -> Mux/136
  P_FV_137/1 -> Mux/137
  P_FV_138/1 -> Mux/138
  P_FV_139/1 -> Mux/139
  P_FV_140/1 -> Mux/140
  P_FV_141/1 -> Mux/141
  P_FV_142/1 -> Mux/142
  P_FV_143/1 -> Mux/143
  P_FV_144/1 -> Mux/144
  P_FV_145/1 -> Mux/145
  P_FV_146/1 -> Mux/146
  P_FV_147/1 -> Mux/147
  P_FV_148/1 -> Mux/148
  P_FV_149/1 -> Mux/149
  P_FV_150/1 -> Mux/150
  P_FV_151/1 -> Mux/151
  P_FV_152/1 -> Mux/152
  P_FV_153/1 -> Mux/153
  P_FV_154/1 -> Mux/154
  P_FV_155/1 -> Mux/155
  P_FV_156/1 -> Mux/156
  P_FV_157/1 -> Mux/157
  P_FV_158/1 -> Mux/158
  P_FV_159/1 -> Mux/159
  P_FV_160/1 -> Mux/160
  P_FV_161/1 -> Mux/161
  P_FV_162/1 -> Mux/162
  P_FV_163/1 -> Mux/163
  P_FV_164/1 -> Mux/164
  P_FV_165/1 -> Mux/165
  P_FV_166/1 -> Mux/166
  P_FV_167/1 -> Mux/167
  P_FV_168/1 -> Mux/168
  P_FV_169/1 -> Mux/169
  P_FV_170/1 -> Mux/170
  P_FV_171/1 -> Mux/171
  P_FV_172/1 -> Mux/172
  P_FV_173/1 -> Mux/173
  P_FV_174/1 -> Mux/174
  P_FV_175/1 -> Mux/175
  P_FV_176/1 -> Mux/176
  P_FV_177/1 -> Mux/177
  P_FV_178/1 -> Mux/178
  P_FV_179/1 -> Mux/179
  P_FV_180/1 -> Mux/180
  P_FV_181/1 -> Mux/181
  P_FV_182/1 -> Mux/182
  P_FV_183/1 -> Mux/183
  P_FV_184/1 -> Mux/184
  P_FV_185/1 -> Mux/185
  P_FV_186/1 -> Mux/186
  P_FV_187/1 -> Mux/187
  P_FV_188/1 -> Mux/188
  P_FV_189/1 -> Mux/189
  P_FV_190/1 -> Mux/190
  P_FV_191/1 -> Mux/191
  P_FV_192/1 -> Mux/192
  P_FV_193/1 -> Mux/193
  P_FV_194/1 -> Mux/194
  P_FV_195/1 -> Mux/195
  P_FV_196/1 -> Mux/196
  P_FV_197/1 -> Mux/197
  P_FV_198/1 -> Mux/198
  P_FV_199/1 -> Mux/199
  P_FV_200/1 -> Mux/200
  P_FV_201/1 -> Mux/201
  P_FV_202/1 -> Mux/202
  P_FV_203/1 -> Mux/203
  P_FV_204/1 -> Mux/204
  P_FV_205/1 -> Mux/205
  P_FV_206/1 -> Mux/206
  P_FV_207/1 -> Mux/207
  P_FV_208/1 -> Mux/208
  P_FV_209/1 -> Mux/209
  P_FV_210/1 -> Mux/210
  P_FV_211/1 -> Mux/211
  P_FV_212/1 -> Mux/212
  P_FV_213/1 -> Mux/213
  P_FV_214/1 -> Mux/214
  P_FV_215/1 -> Mux/215
  P_FV_216/1 -> Mux/216
  P_FV_217/1 -> Mux/217
  P_FV_218/1 -> Mux/218
  P_FV_219/1 -> Mux/219
  P_FV_220/1 -> Mux/220
  P_FV_221/1 -> Mux/221
  P_FV_222/1 -> Mux/222
  P_FV_223/1 -> Mux/223
  P_FV_224/1 -> Mux/224
  P_FV_225/1 -> Mux/225
  P_FV_226/1 -> Mux/226
  P_FV_227/1 -> Mux/227
  P_FV_228/1 -> Mux/228
  P_FV_229/1 -> Mux/229
  P_FV_230/1 -> Mux/230
  P_FV_231/1 -> Mux/231
  P_FV_232/1 -> Mux/232
  P_FV_233/1 -> Mux/233
  P_FV_234/1 -> Mux/234
  P_FV_235/1 -> Mux/235
  P_FV_236/1 -> Mux/236
  P_FV_237/1 -> Mux/237
  P_FV_238/1 -> Mux/238
  P_FV_239/1 -> Mux/239
  P_FV_240/1 -> Mux/240
  P_FV_241/1 -> Mux/241
  P_FV_242/1 -> Mux/242
  P_FV_243/1 -> Mux/243
  P_FV_244/1 -> Mux/244
  P_FV_245/1 -> Mux/245
  P_FV_246/1 -> Mux/246
  P_FV_247/1 -> Mux/247
  P_FV_248/1 -> Mux/248
  P_FV_249/1 -> Mux/249
  P_FV_250/1 -> Mux/250
  P_FV_251/1 -> Mux/251
  P_FV_252/1 -> Mux/252
  P_FV_253/1 -> Mux/253
  P_FV_254/1 -> Mux/254
  P_FV_255/1 -> Mux/255
  P_FV_256/1 -> Mux/256
  P_FV_257/1 -> Mux/257
  P_FV_258/1 -> Mux/258
  P_FV_259/1 -> Mux/259
  P_FV_260/1 -> Mux/260
  P_FV_261/1 -> Mux/261
  P_FV_262/1 -> Mux/262
  P_FV_263/1 -> Mux/263
  P_FV_264/1 -> Mux/264
  P_FV_265/1 -> Mux/265
  P_FV_266/1 -> Mux/266
  P_FV_267/1 -> Mux/267
  P_FV_268/1 -> Mux/268
  P_FV_269/1 -> Mux/269
  P_FV_270/1 -> Mux/270
  P_FV_271/1 -> Mux/271
  P_FV_272/1 -> Mux/272
  P_FV_273/1 -> Mux/273
  P_FV_274/1 -> Mux/274
  P_FV_275/1 -> Mux/275
  P_FV_276/1 -> Mux/276
  P_FV_277/1 -> Mux/277
  P_FV_278/1 -> Mux/278
  P_FV_279/1 -> Mux/279
  P_FV_280/1 -> Mux/280
  P_FV_281/1 -> Mux/281
  P_FV_282/1 -> Mux/282
  P_FV_283/1 -> Mux/283
  P_FV_284/1 -> Mux/284
  P_FV_285/1 -> Mux/285
  P_FV_286/1 -> Mux/286
  P_FV_287/1 -> Mux/287
  P_FV_288/1 -> Mux/288
  P_FV_289/1 -> Mux/289
  P_FV_290/1 -> Mux/290
  P_FV_291/1 -> Mux/291
  P_FV_292/1 -> Mux/292
  P_FV_293/1 -> Mux/293
  P_FV_294/1 -> Mux/294
  P_FV_295/1 -> Mux/295
  P_FV_296/1 -> Mux/296
  P_FV_297/1 -> Mux/297
  P_FV_298/1 -> Mux/298
  P_FV_299/1 -> Mux/299
  P_FV_300/1 -> Mux/300

== system xEMU_SimulationModel3_rule1/Battery (BAT)_mittel/Battery/Thermal/Coolings ==
  T_FV : Inport
  CoolAdder : Subsystem
  P_FV : Outport
  wires:
  CoolAdder/1(P_FV) -> P_FV/1
